simulink model "Test3C120Board_Leds"  (Simulink 6.4)
settings: Solver=ode45  SolverMode=SingleTasking  StartTime=0.0  StopTime=100000.0  FixedStep=1  RelTol=1e-3
InitFcn:
  | %% DSPBuilder Start
  | alt_dspbuilder_update_model(bdroot)
  | %% DSPBuilder End
undefined symbols (not defined in the file): Pin_AB15, Pin_AC14, Pin_AC19, Pin_AD14, Pin_AD18, Pin_AF25, Pin_AG23, Pin_G20
libraries: allblocks_alteradspbuilder2 x19, Cyclone_III_EP3C120_alteradspbuilder2 x14
settings Model: Creator=lkong  LastModifiedBy=lkong
settings DataIOCC: SignalLoggingName=sigsOut
settings OptimizationCC: InlineInvariantSignals=on
settings DebuggingCC: SolverPrmCheckMsg=none  StrictBusMsg=None
settings HardwareCC: TargetUnknown=on
settings GRTTargetCC: ModelReferenceCompliant=off  MatFileLogging=off

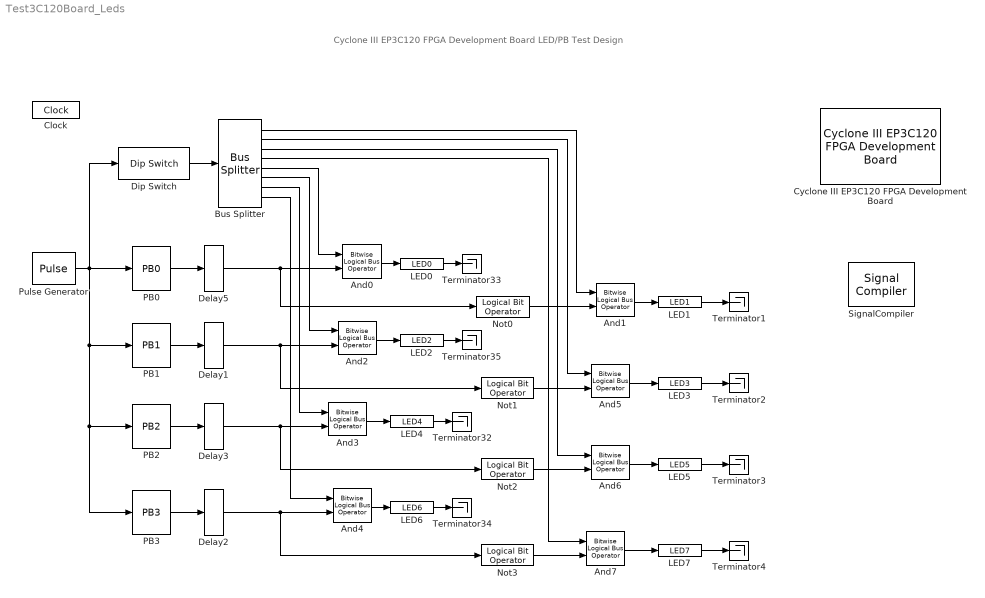
== system Test3C120Board_Leds ==
  note: Cyclone III EP3C120 FPGA Development Board LED/PB Test Design
  And{0..7} (8 alike) : allblocks_alteradspbuilder2/Bitwise Logical Bus Operator  BusType=Inferred  bwl=1  bwr=0  LogicalOperator=AND  pipeline_display=0
  Bus Splitter : allblocks_alteradspbuilder2/Bus Splitter  BusType=Signed Integer  bwl=8  bwr=0  pipeline_display=0
  Clock : allblocks_alteradspbuilder2/Clock  ClockPeriod=10  ClockPeriodUnit=ns  SampleTime=1  SimulationStartCycle=5  PhaseOffset=0  Reset=aclr  ResetType=Active Low  Export=off
  Cyclone III EP3C120 FPGA Development Board : Cyclone_III_EP3C120_alteradspbuilder2/Cyclone III EP3C120 FPGA Development Board  ClockPinIn=Pin_AH15  GlobalResetPin=Pin_T21  device=EP3C120F780C7
  Delay1 : allblocks_alteradspbuilder2/Delay  pipeline=1  pipeline_display=1  ClockPhase=1  use_ena=off  use_sclr=off  allowFloatingPointOverride=on  logOutputs=off  logFile=d:\ws80\workspace\Documentation\DesignExamples\Demos\Board\CycloneIII_DSPBoard_3C120\tb_Test3C120Board_Leds\Test3C120Board%5FLeds_Delay1.fixedpointlog  use_init=off  reset_value=1
  Delay2 : allblocks_alteradspbuilder2/Delay  pipeline=1  pipeline_display=1  ClockPhase=1  use_ena=off  use_sclr=off  allowFloatingPointOverride=on  logOutputs=off  logFile=d:\ws80\workspace\Documentation\DesignExamples\Demos\Board\CycloneIII_DSPBoard_3C120\tb_Test3C120Board_Leds\Test3C120Board%5FLeds_Delay2.fixedpointlog  use_init=off  reset_value=1
  Delay3 : allblocks_alteradspbuilder2/Delay  pipeline=1  pipeline_display=1  ClockPhase=1  use_ena=off  use_sclr=off  allowFloatingPointOverride=on  logOutputs=off  logFile=d:\ws80\workspace\Documentation\DesignExamples\Demos\Board\CycloneIII_DSPBoard_3C120\tb_Test3C120Board_Leds\Test3C120Board%5FLeds_Delay3.fixedpointlog  use_init=off  reset_value=1
  Delay5 : allblocks_alteradspbuilder2/Delay  pipeline=1  pipeline_display=1  ClockPhase=1  use_ena=off  use_sclr=off  allowFloatingPointOverride=on  logOutputs=off  logFile=d:\ws80\workspace\Documentation\DesignExamples\Demos\Board\CycloneIII_DSPBoard_3C120\tb_Test3C120Board_Leds\Test3C120Board%5FLeds_Delay5.fixedpointlog  use_init=off  reset_value=1
  Dip Switch : Cyclone_III_EP3C120_alteradspbuilder2/Dip Switch  iofile=d:\ws80\workspace\Documentation\DesignExamples\Demos\Board\CycloneIII_DSPBoard_3C120\tb_Test3C120Board_Leds\Test3C120Board%5FLeds_Dip+Switch.salt  externalType=Inferred  SpecifyClock=off  location=Pin_AC14,Pin_AD18,Pin_AG23,Pin_AC19,Pin_AD14,Pin_G20,Pin_AB15,Pin_AF25
  LED0 : Cyclone_III_EP3C120_alteradspbuilder2/LED0  iofile=d:\ws80\workspace\Documentation\DesignExamples\Demos\Board\CycloneIII_DSPBoard_3C120\tb_Test3C120Board_Leds\Test3C120Board%5FLeds_LED0.capture  externalType=Inferred  location=Pin_AD15
  LED1 : Cyclone_III_EP3C120_alteradspbuilder2/LED1  iofile=d:\ws80\workspace\Documentation\DesignExamples\Demos\Board\CycloneIII_DSPBoard_3C120\tb_Test3C120Board_Leds\Test3C120Board%5FLeds_LED1.capture  externalType=Inferred  location=Pin_AE20
  LED2 : Cyclone_III_EP3C120_alteradspbuilder2/LED2  iofile=d:\ws80\workspace\Documentation\DesignExamples\Demos\Board\CycloneIII_DSPBoard_3C120\tb_Test3C120Board_Leds\Test3C120Board%5FLeds_LED2.capture  externalType=Inferred  location=Pin_AF18
  LED3 : Cyclone_III_EP3C120_alteradspbuilder2/LED3  iofile=d:\ws80\workspace\Documentation\DesignExamples\Demos\Board\CycloneIII_DSPBoard_3C120\tb_Test3C120Board_Leds\Test3C120Board%5FLeds_LED3.capture  externalType=Inferred  location=Pin_AD19
  LED4 : Cyclone_III_EP3C120_alteradspbuilder2/LED4  iofile=d:\ws80\workspace\Documentation\DesignExamples\Demos\Board\CycloneIII_DSPBoard_3C120\tb_Test3C120Board_Leds\Test3C120Board%5FLeds_LED4.capture  externalType=Inferred  location=Pin_AE15
  LED5 : Cyclone_III_EP3C120_alteradspbuilder2/LED5  iofile=d:\ws80\workspace\Documentation\DesignExamples\Demos\Board\CycloneIII_DSPBoard_3C120\tb_Test3C120Board_Leds\Test3C120Board%5FLeds_LED5.capture  externalType=Inferred  location=Pin_AC17
  LED6 : Cyclone_III_EP3C120_alteradspbuilder2/LED6  iofile=d:\ws80\workspace\Documentation\DesignExamples\Demos\Board\CycloneIII_DSPBoard_3C120\tb_Test3C120Board_Leds\Test3C120Board%5FLeds_LED6.capture  externalType=Inferred  location=Pin_AG19
  LED7 : Cyclone_III_EP3C120_alteradspbuilder2/LED7  iofile=d:\ws80\workspace\Documentation\DesignExamples\Demos\Board\CycloneIII_DSPBoard_3C120\tb_Test3C120Board_Leds\Test3C120Board%5FLeds_LED7.capture  externalType=Inferred  location=Pin_AF19
  Not{0..3} (4 alike) : allblocks_alteradspbuilder2/Logical Bit Operator  LogicalOperator=NOT  user_inputs=2  pipeline_display=0
  PB0 : Cyclone_III_EP3C120_alteradspbuilder2/PB0  iofile=d:\ws80\workspace\Documentation\DesignExamples\Demos\Board\CycloneIII_DSPBoard_3C120\tb_Test3C120Board_Leds\Test3C120Board%5FLeds_PB0.salt  externalType=Inferred  SpecifyClock=off  location=Pin_AD7
  PB1 : Cyclone_III_EP3C120_alteradspbuilder2/PB1  iofile=d:\ws80\workspace\Documentation\DesignExamples\Demos\Board\CycloneIII_DSPBoard_3C120\tb_Test3C120Board_Leds\Test3C120Board%5FLeds_PB1.salt  externalType=Inferred  SpecifyClock=off  location=Pin_AC12
  PB2 : Cyclone_III_EP3C120_alteradspbuilder2/PB2  iofile=d:\ws80\workspace\Documentation\DesignExamples\Demos\Board\CycloneIII_DSPBoard_3C120\tb_Test3C120Board_Leds\Test3C120Board%5FLeds_PB2.salt  externalType=Inferred  SpecifyClock=off  location=Pin_AH3
  PB3 : Cyclone_III_EP3C120_alteradspbuilder2/PB3  iofile=d:\ws80\workspace\Documentation\DesignExamples\Demos\Board\CycloneIII_DSPBoard_3C120\tb_Test3C120Board_Leds\Test3C120Board%5FLeds_PB3.salt  externalType=Inferred  SpecifyClock=off  location=Pin_AA12
  Pulse Generator : DiscretePulseGenerator  Period=20000  PulseWidth=2
  SignalCompiler : allblocks_alteradspbuilder2/Signal Compiler  DeviceFamily=Cyclone III  DeviceName=EP3C120F780C7  EnableSignalTap=on  SignalTapDepth=512  UseBoardBlock=on  StpUseDefaultClock=on  StpClock=Clock  ExportDir=D:\MATLAB\R2006a\work
  Terminator{1..4,32..35} (8 alike) : Terminator
  wires:
  PB0/1 -> Delay5/1
  PB1/1 -> Delay1/1
  PB2/1 -> Delay3/1
  PB3/1 -> Delay2/1
  Delay2/1 -> Not3/1, And4/2
  Delay3/1 -> Not2/1, And3/2
  Delay1/1 -> Not1/1, And2/2
  Delay5/1 -> Not0/1, And0/2
  LED4/1 -> Terminator32/1
  LED0/1 -> Terminator33/1
  LED6/1 -> Terminator34/1
  LED2/1 -> Terminator35/1
  Pulse Generator/1 -> PB3/1, PB2/1, PB1/1, PB0/1, Dip Switch/1
  LED1/1 -> Terminator1/1
  LED3/1 -> Terminator2/1
  LED5/1 -> Terminator3/1
  LED7/1 -> Terminator4/1
  Dip Switch/1 -> Bus Splitter/1
  And0/1 -> LED0/1
  Not0/1 -> And1/2
  And1/1 -> LED1/1
  And2/1 -> LED2/1
  And3/1 -> LED4/1
  And4/1 -> LED6/1
  Bus Splitter/1 -> And1/1
  And5/1 -> LED3/1
  Not1/1 -> And5/2
  Bus Splitter/2 -> And5/1
  And6/1 -> LED5/1
  Not2/1 -> And6/2
  And7/1 -> LED7/1
  Bus Splitter/3 -> And6/1
  Bus Splitter/4 -> And7/1
  Not3/1 -> And7/2
  Bus Splitter/8 -> And4/1
  Bus Splitter/7 -> And3/1
  Bus Splitter/6 -> And2/1
  Bus Splitter/5 -> And0/1
